simulink model "Supervisory_Control_System"  (R2021a)
settings: Solver=VariableStepAuto  StartTime=0.0  StopTime=10.0  RelTol=1e-3
libraries: simulink x3
settings Model: Creator=shind  LastModifiedBy=shind

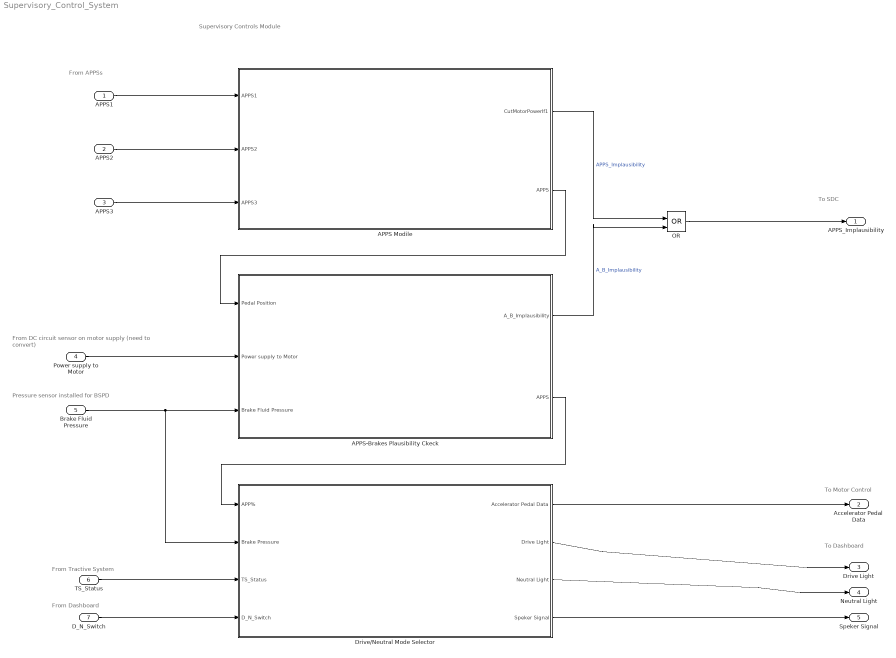
== system Supervisory_Control_System ==
  note: Supervisory Controls Module
  note: From APPSs
  note: To SDC
  note: Pressure sensor installed for
      | BSPD
  note: From DC circuit sensor on motor
      | supply (need to convert)
  note: From Tractive System
  note: From Dashboard
  note: To Motor Control
  note: To Dashboard
  APPS1 : Inport
  APPS2 : Inport  Port=2
  APPS3 : Inport  Port=3
  Power supply to Motor : Inport  Port=4
  Brake Fluid Pressure : Inport  Port=5
  TS_Status : Inport  Port=6
  D_N_Switch : Inport  Port=7
  APPS Modile : Subsystem
  APPS-Brakes Plausibility Ckeck : Subsystem
  Drive/Neutral Mode Selector : Subsystem
  OR : Logic  Operator=OR  IconShape=distinctive  AllPortsSameDT=off  OutDataTypeStr=boolean
  APPS_Implausibility : Outport
  Accelerator Pedal Data : Outport  Port=2
  Drive Light : Outport  Port=3
  Neutral Light : Outport  Port=4
  Speker Signal : Outport  Port=5
  wires:
  APPS2/1 -> APPS Modile/2(APPS2)
  APPS1/1 -> APPS Modile/1(APPS1)
  APPS3/1 -> APPS Modile/3(APPS3)
  APPS Modile/1(CutMotorPowerIf1) -> OR/1  "APPS_Implausibility"
  Power supply to Motor/1 -> APPS-Brakes Plausibility Ckeck/2(Power supply to Motor)
  APPS-Brakes Plausibility Ckeck/1(A_B_Implausibility) -> OR/2  "A_B_Implausibility"
  TS_Status/1 -> Drive/Neutral Mode Selector/3(TS_Status)
  Brake Fluid Pressure/1 -> APPS-Brakes Plausibility Ckeck/3(Brake Fluid Pressure), Drive/Neutral Mode Selector/2(Brake Pressure)
  D_N_Switch/1 -> Drive/Neutral Mode Selector/4(D_N_Switch)
  Drive/Neutral Mode Selector/2(Drive Light) -> Drive Light/1
  Drive/Neutral Mode Selector/3(Neutral Light) -> Neutral Light/1
  Drive/Neutral Mode Selector/1(Accelerator Pedal Data) -> Accelerator Pedal Data/1
  Drive/Neutral Mode Selector/4(Speker Signal) -> Speker Signal/1
  APPS Modile/2(APPS) -> APPS-Brakes Plausibility Ckeck/1(Pedal Position)
  APPS-Brakes Plausibility Ckeck/2(APPS) -> Drive/Neutral Mode Selector/1(APP%)
  OR/1 -> APPS_Implausibility/1

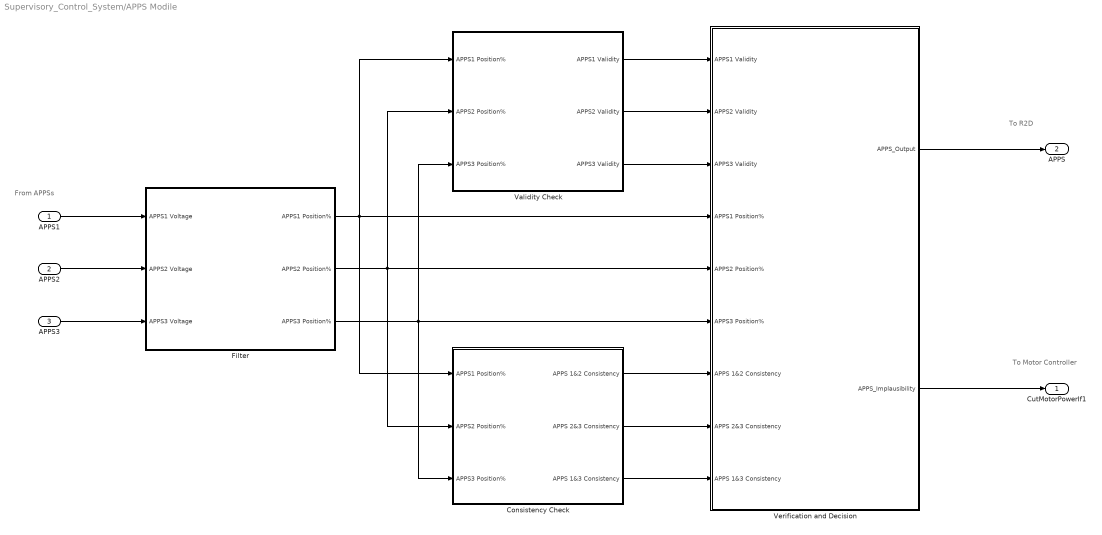
== system Supervisory_Control_System/APPS Modile ==
  note: From APPSs
  note: To Motor Controller
  note: To R2D
  APPS1 : Inport
  APPS2 : Inport  Port=2
  APPS3 : Inport  Port=3
  Consistency Check : Subsystem
  Filter : Subsystem
  Validity Check : Subsystem
  Verification and Decision : Subsystem
  CutMotorPowerIf1 : Outport
  APPS : Outport  Port=2
  wires:
  Verification and Decision/2(APPS_Implausibility) -> CutMotorPowerIf1/1
  APPS2/1 -> Filter/2(APPS2 Voltage)
  Consistency Check/2(APPS 2&3 Consistency) -> Verification and Decision/8(APPS 2&3 Consistency)
  Validity Check/2(APPS2 Validity) -> Verification and Decision/2(APPS2 Validity)
  Filter/1(APPS1 Position%) -> Consistency Check/1(APPS1 Position%), Validity Check/1(APPS1 Position%), Verification and Decision/4(APPS1 Position%)
  Consistency Check/1(APPS 1&2 Consistency) -> Verification and Decision/7(APPS 1&2 Consistency)
  Filter/3(APPS3 Position%) -> Consistency Check/3(APPS3 Position%), Validity Check/3(APPS3 Position%), Verification and Decision/6(APPS3 Position%)
  Validity Check/1(APPS1 Validity) -> Verification and Decision/1(APPS1 Validity)
  Validity Check/3(APPS3 Validity) -> Verification and Decision/3(APPS3 Validity)
  APPS1/1 -> Filter/1(APPS1 Voltage)
  Verification and Decision/1(APPS_Output) -> APPS/1
  APPS3/1 -> Filter/3(APPS3 Voltage)
  Filter/2(APPS2 Position%) -> Consistency Check/2(APPS2 Position%), Validity Check/2(APPS2 Position%), Verification and Decision/5(APPS2 Position%)
  Consistency Check/3(APPS 1&3 Consistency) -> Verification and Decision/9(APPS 1&3 Consistency)

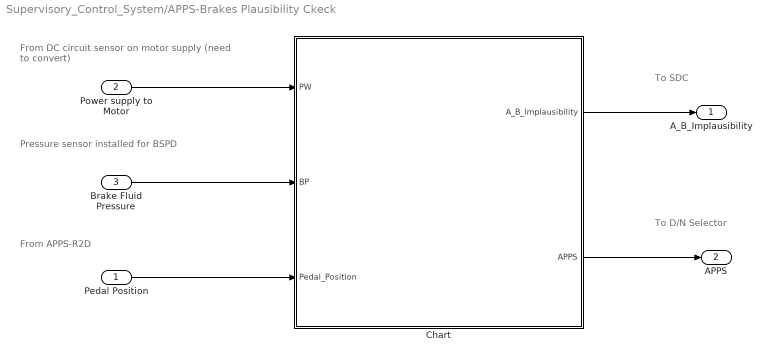
== system Supervisory_Control_System/APPS-Brakes Plausibility Ckeck ==
  note: From DC circuit sensor on motor
      | supply (need to convert)
  note: From APPS-R2D
  note: Pressure sensor installed for
      | BSPD
  note: To SDC
  note: To D/N Selector
  Pedal Position : Inport
  Power supply to Motor : Inport  Port=2
  Brake Fluid Pressure : Inport  Port=3
  Chart : Stateflow chart  TreatAsAtomicUnit=on
  A_B_Implausibility : Outport
  APPS : Outport  Port=2
  wires:
  Power supply to Motor/1 -> Chart/1(PW)
  Brake Fluid Pressure/1 -> Chart/2(BP)
  Pedal Position/1 -> Chart/3(Pedal_Position)
  Chart/1(A_B_Implausibility) -> A_B_Implausibility/1
  Chart/2(APPS) -> APPS/1

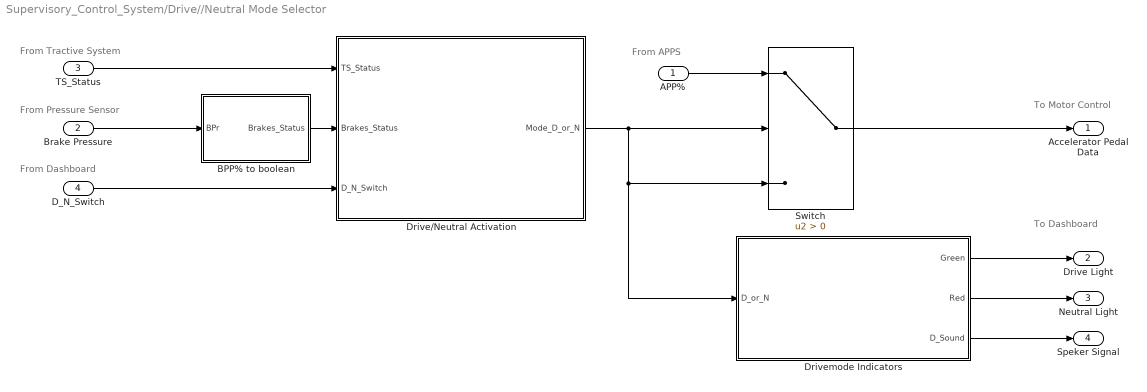
== system Supervisory_Control_System/Drive//Neutral Mode Selector ==
  note: To Motor Control
  note: From Pressure Sensor
  note: From APPS
  note: To Dashboard
  note: From Dashboard
  note: From Tractive System
  APP% : Inport
  Brake Pressure : Inport  Port=2
  TS_Status : Inport  Port=3
  D_N_Switch : Inport  Port=4
  BPP% to boolean : Stateflow chart  TreatAsAtomicUnit=on
  Drive/Neutral Activation : Stateflow chart  TreatAsAtomicUnit=on
  Drivemode Indicators : Stateflow chart  TreatAsAtomicUnit=on
  Switch : Switch  Criteria=u2 > Threshold
  Accelerator Pedal Data : Outport
  Drive Light : Outport  Port=2
  Neutral Light : Outport  Port=3
  Speker Signal : Outport  Port=4
  wires:
  D_N_Switch/1 -> Drive/Neutral Activation/3(D_N_Switch)
  APP%/1 -> Switch/1
  Drive/Neutral Activation/1(Mode_D_or_N) -> Switch/2, Drivemode Indicators/1(D_or_N), Switch/3
  Brake Pressure/1 -> BPP% to boolean/1(BPr)
  BPP% to boolean/1(Brakes_Status) -> Drive/Neutral Activation/2(Brakes_Status)
  Drivemode Indicators/3(D_Sound) -> Speker Signal/1
  Drivemode Indicators/1(Green) -> Drive Light/1
  TS_Status/1 -> Drive/Neutral Activation/1(TS_Status)
  Drivemode Indicators/2(Red) -> Neutral Light/1
  Switch/1 -> Accelerator Pedal Data/1

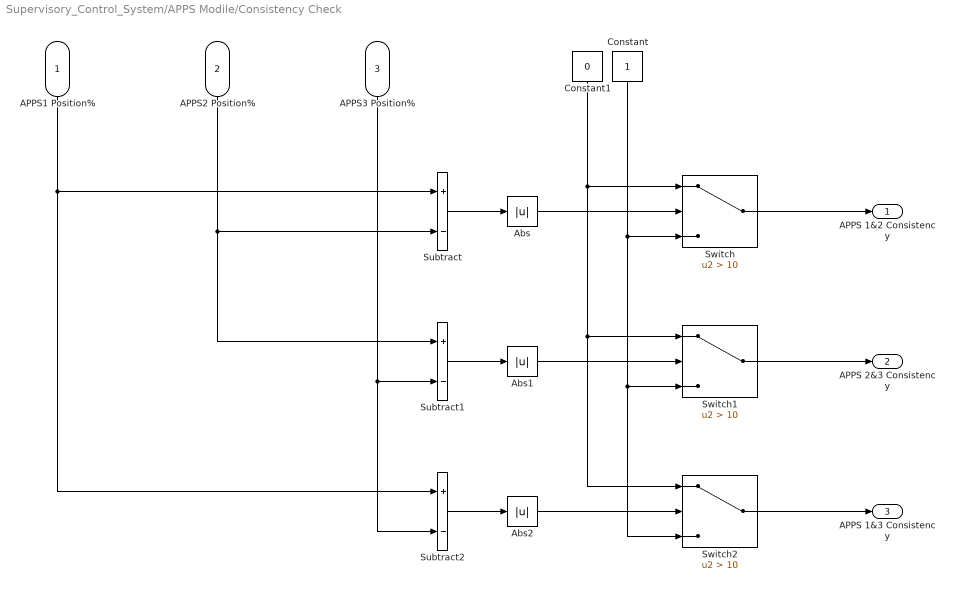
== system Supervisory_Control_System/APPS Modile/Consistency Check ==
  APPS1 Position% : Inport
  APPS2 Position% : Inport  Port=2
  APPS3 Position% : Inport  Port=3
  Abs : Abs
  Abs1 : Abs
  Abs2 : Abs
  Constant : Constant
  Constant1 : Constant  Value=0
  Subtract : Sum  Inputs=+-
  Subtract1 : Sum  Inputs=+-
  Subtract2 : Sum  Inputs=+-
  Switch : Switch  Criteria=u2 > Threshold  Threshold=10
  Switch1 : Switch  Criteria=u2 > Threshold  Threshold=10
  Switch2 : Switch  Criteria=u2 > Threshold  Threshold=10
  APPS 1&2 Consistency : Outport
  APPS 2&3 Consistency : Outport  Port=2
  APPS 1&3 Consistency : Outport  Port=3
  wires:
  Subtract/1 -> Abs/1
  Subtract1/1 -> Abs1/1
  Subtract2/1 -> Abs2/1
  APPS1 Position%/1 -> Subtract/1, Subtract2/1
  APPS2 Position%/1 -> Subtract/2, Subtract1/1
  APPS3 Position%/1 -> Subtract1/2, Subtract2/2
  Abs/1 -> Switch/2
  Constant1/1 -> Switch/1, Switch1/1, Switch2/1
  Constant/1 -> Switch2/3, Switch1/3, Switch/3
  Abs1/1 -> Switch1/2
  Abs2/1 -> Switch2/2
  Switch/1 -> APPS 1&2 Consistency/1
  Switch1/1 -> APPS 2&3 Consistency/1
  Switch2/1 -> APPS 1&3 Consistency/1

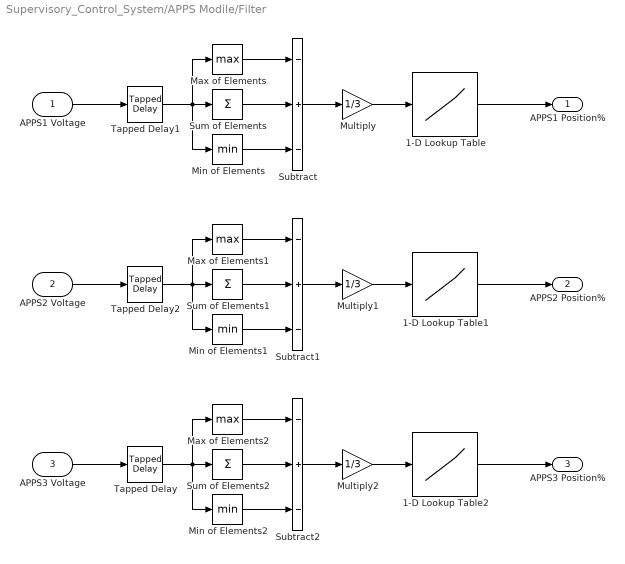
== system Supervisory_Control_System/APPS Modile/Filter ==
  APPS1 Voltage : Inport
  APPS2 Voltage : Inport  Port=2
  APPS3 Voltage : Inport  Port=3
  1-D Lookup Table : Lookup_n-D  NumberOfTableDimensions=1  BreakpointsForDimension1=[-5:5]  Table=tanh([-5:5])  InternalRulePriority=Speed  RndMeth=Simplest  InputSameDT=on
  1-D Lookup Table1 : Lookup_n-D  NumberOfTableDimensions=1  BreakpointsForDimension1=[-5:5]  Table=tanh([-5:5])  InternalRulePriority=Speed  RndMeth=Simplest  InputSameDT=on
  1-D Lookup Table2 : Lookup_n-D  NumberOfTableDimensions=1  BreakpointsForDimension1=[-5:5]  Table=tanh([-5:5])  InternalRulePriority=Speed  RndMeth=Simplest  InputSameDT=on
  Max of Elements : MinMax  Function=max
  Max of Elements1 : MinMax  Function=max
  Max of Elements2 : MinMax  Function=max
  Min of Elements : MinMax
  Min of Elements1 : MinMax
  Min of Elements2 : MinMax
  Multiply : Gain  Gain=1/3
  Multiply1 : Gain  Gain=1/3
  Multiply2 : Gain  Gain=1/3
  Subtract : Sum  Inputs=-+-
  Subtract1 : Sum  Inputs=-+-
  Subtract2 : Sum  Inputs=-+-
  Sum of Elements : Sum  Inputs=+
  Sum of Elements1 : Sum  Inputs=+
  Sum of Elements2 : Sum  Inputs=+
  Tapped Delay : simulink/Discrete/Tapped Delay  vinit=0.0  samptime=-1  NumDelays=5  DelayOrder=Oldest  includeCurrent=off
  Tapped Delay1 : simulink/Discrete/Tapped Delay  vinit=0.0  samptime=-1  NumDelays=5  DelayOrder=Oldest  includeCurrent=off
  Tapped Delay2 : simulink/Discrete/Tapped Delay  vinit=0.0  samptime=-1  NumDelays=5  DelayOrder=Oldest  includeCurrent=off
  APPS1 Position% : Outport
  APPS2 Position% : Outport  Port=2
  APPS3 Position% : Outport  Port=3
  wires:
  Multiply2/1 -> 1-D Lookup Table2/1
  1-D Lookup Table2/1 -> APPS3 Position%/1
  Multiply/1 -> 1-D Lookup Table/1
  APPS2 Voltage/1 -> Tapped Delay2/1
  Max of Elements/1 -> Subtract/1
  Subtract2/1 -> Multiply2/1
  Sum of Elements/1 -> Subtract/2
  Max of Elements2/1 -> Subtract2/1
  Sum of Elements2/1 -> Subtract2/2
  Sum of Elements1/1 -> Subtract1/2
  Subtract1/1 -> Multiply1/1
  Subtract/1 -> Multiply/1
  Min of Elements1/1 -> Subtract1/3
  1-D Lookup Table1/1 -> APPS2 Position%/1
  Min of Elements2/1 -> Subtract2/3
  APPS1 Voltage/1 -> Tapped Delay1/1
  Max of Elements1/1 -> Subtract1/1
  Min of Elements/1 -> Subtract/3
  APPS3 Voltage/1 -> Tapped Delay/1
  Multiply1/1 -> 1-D Lookup Table1/1
  Tapped Delay2/1 -> Sum of Elements1/1, Max of Elements1/1, Min of Elements1/1
  Tapped Delay1/1 -> Max of Elements/1, Sum of Elements/1, Min of Elements/1
  Tapped Delay/1 -> Sum of Elements2/1, Max of Elements2/1, Min of Elements2/1
  1-D Lookup Table/1 -> APPS1 Position%/1

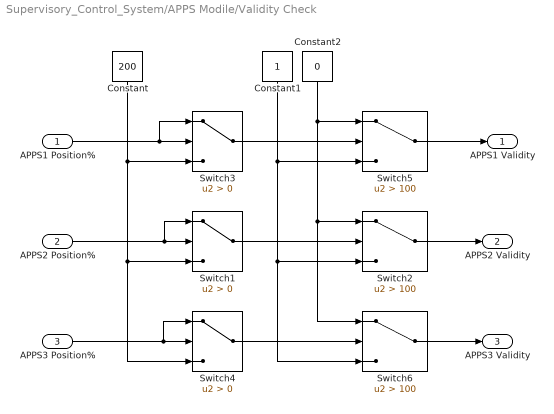
== system Supervisory_Control_System/APPS Modile/Validity Check ==
  APPS1 Position% : Inport
  APPS2 Position% : Inport  Port=2
  APPS3 Position% : Inport  Port=3
  Constant : Constant  Value=200
  Constant1 : Constant
  Constant2 : Constant  Value=0
  Switch1 : Switch  Criteria=u2 > Threshold
  Switch2 : Switch  Criteria=u2 > Threshold  Threshold=100
  Switch3 : Switch  Criteria=u2 > Threshold
  Switch4 : Switch  Criteria=u2 > Threshold
  Switch5 : Switch  Criteria=u2 > Threshold  Threshold=100
  Switch6 : Switch  Criteria=u2 > Threshold  Threshold=100
  APPS1 Validity : Outport
  APPS2 Validity : Outport  Port=2
  APPS3 Validity : Outport  Port=3
  wires:
  Switch5/1 -> APPS1 Validity/1
  APPS1 Position%/1 -> Switch3/1, Switch3/2
  Switch3/1 -> Switch5/2
  Switch1/1 -> Switch2/2
  APPS2 Position%/1 -> Switch1/2, Switch1/1
  Switch2/1 -> APPS2 Validity/1
  Switch6/1 -> APPS3 Validity/1
  APPS3 Position%/1 -> Switch4/1, Switch4/2
  Switch4/1 -> Switch6/2
  Constant/1 -> Switch3/3, Switch1/3, Switch4/3
  Constant1/1 -> Switch6/3, Switch2/3, Switch5/3
  Constant2/1 -> Switch6/1, Switch2/1, Switch5/1

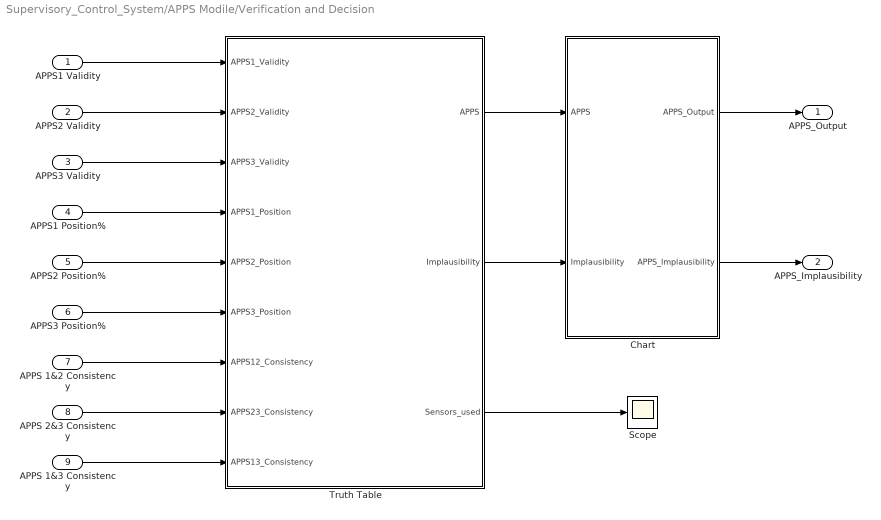
== system Supervisory_Control_System/APPS Modile/Verification and Decision ==
  APPS1 Validity : Inport
  APPS2 Validity : Inport  Port=2
  APPS3 Validity : Inport  Port=3
  APPS1 Position% : Inport  Port=4
  APPS2 Position% : Inport  Port=5
  APPS3 Position% : Inport  Port=6
  APPS 1&2 Consistency : Inport  Port=7
  APPS 2&3 Consistency : Inport  Port=8
  APPS 1&3 Consistency : Inport  Port=9
  Chart : Stateflow chart  TreatAsAtomicUnit=on
  Scope : Scope
  Truth Table : Truth Table  TreatAsAtomicUnit=on
  APPS_Output : Outport
  APPS_Implausibility : Outport  Port=2
  wires:
  APPS1 Validity/1 -> Truth Table/1(APPS1_Validity)
  APPS2 Validity/1 -> Truth Table/2(APPS2_Validity)
  APPS3 Validity/1 -> Truth Table/3(APPS3_Validity)
  APPS1 Position%/1 -> Truth Table/4(APPS1_Position)
  APPS2 Position%/1 -> Truth Table/5(APPS2_Position)
  APPS3 Position%/1 -> Truth Table/6(APPS3_Position)
  APPS 1&2 Consistency/1 -> Truth Table/7(APPS12_Consistency)
  APPS 2&3 Consistency/1 -> Truth Table/8(APPS23_Consistency)
  APPS 1&3 Consistency/1 -> Truth Table/9(APPS13_Consistency)
  Truth Table/3(Sensors_used) -> Scope/1
  Truth Table/1(APPS) -> Chart/1(APPS)
  Truth Table/2(Implausibility) -> Chart/2(Implausibility)
  Chart/1(APPS_Output) -> APPS_Output/1
  Chart/2(APPS_Implausibility) -> APPS_Implausibility/1

== stateflow chart Supervisory_Control_System/Drive//Neutral Mode Selector/Drivemode Indicators ==
  state Neutral
    entry:
    Red=1;
    Green=0;
  state Drive
    entry:
    Red=0;
    Green=1;
    state sound_start
      entry:
      D_Sound=1;
    state sound_stop
      entry:
      D_Sound=0;
    (default) -> sound_start
    sound_start -> sound_stop : after(2,sec)
  (default) -> Neutral
  Neutral -> Drive : [D_or_N==1]
  Drive -> Neutral : [D_or_N==0]
  data: D_or_N input; Green output; Red output; D_Sound output

== stateflow chart Supervisory_Control_System/APPS-Brakes Plausibility Ckeck/Chart ==
  state Normal
    entry:
    A_B_Implausibility=0;
    APPS=Pedal_Position;
  state APPS_Brake_Implausible
    entry:
    A_B_Implausibility=1;
    APPS=0;
  state Time_Check
  (default) -> Normal
  Normal -> Time_Check : [BP>=30 && PW>=5000]
  Time_Check -> APPS_Brake_Implausible [order 1] : after(500,msec)
  Time_Check -> Normal [order 2] : [BP<30 || PW<5000]
  APPS_Brake_Implausible -> Normal : [Pedal_Position==0]
  data: A_B_Implausibility output; PW input; BP input; Pedal_Position input; APPS output

== matlab function Supervisory_Control_System/APPS Modile/Verification and Decision/Truth Table ==
  data: APPS1_Validity input; APPS2_Validity input double; APPS3_Validity input double; APPS1_Position input double; APPS2_Position input double; APPS3_Position input double; APPS12_Consistency input double; APPS23_Consistency input double; APPS13_Consistency input double; APPS output double; Implausibility output double; Sensors_used output double
function [APPS, Implausibility, Sensors_used] = fcn(APPS1_Validity, APPS2_Validity, APPS3_Validity, APPS1_Position, APPS2_Position, APPS3_Position, APPS12_Consistency, APPS23_Consistency, APPS13_Consistency)

aVarTruthTableCondition_1 = false;
aVarTruthTableCondition_2 = false;
aVarTruthTableCondition_3 = false;
aVarTruthTableCondition_4 = false;
aVarTruthTableCondition_5 = false;
aVarTruthTableCondition_6 = false;


% 1 Validity

aVarTruthTableCondition_1 = logical(APPS1_Validity==1);

% 2 Validity

aVarTruthTableCondition_2 = logical(APPS2_Validity==1);

% 3 Validity

aVarTruthTableCondition_3 = logical(APPS3_Validity==1);

% 12 Consistency

aVarTruthTableCondition_4 = logical(APPS12_Consistency==1);

% 23 Consistency

aVarTruthTableCondition_5 = logical(APPS23_Consistency==1);

% 13 Consistency

aVarTruthTableCondition_6 = logical(APPS13_Consistency==1);

if (aVarTruthTableCondition_1 && aVarTruthTableCondition_2 && aVarTruthTableCondition_3 && aVarTruthTableCondition_4 && aVarTruthTableCondition_5 && aVarTruthTableCondition_6)
    aFcnTruthTableAction_1();
elseif (aVarTruthTableCondition_1 && aVarTruthTableCondition_2 && ~aVarTruthTableCondition_3 && aVarTruthTableCondition_4)
    aFcnTruthTableAction_2();
elseif (aVarTruthTableCondition_1 && aVarTruthTableCondition_2 && aVarTruthTableCondition_3 && aVarTruthTableCondition_4 && ~aVarTruthTableCondition_5)
    aFcnTruthTableAction_2();
elseif (aVarTruthTableCondition_1 && aVarTruthTableCondition_2 && aVarTruthTableCondition_3 && aVarTruthTableCondition_4 && ~aVarTruthTableCondition_6)
    aFcnTruthTableAction_2();
elseif (~aVarTruthTableCondition_1 && aVarTruthTableCondition_2 && aVarTruthTableCondition_3 && aVarTruthTableCondition_5)
    aFcnTruthTableAction_3();
elseif (aVarTruthTableCondition_1 && aVarTruthTableCondition_2 && aVarTruthTableCondition_3 && ~aVarTruthTableCondition_4 && aVarTruthTableCondition_5)
    aFcnTruthTableAction_3();
elseif (aVarTruthTableCondition_1 && ~aVarTruthTableCondition_2 && aVarTruthTableCondition_3 && aVarTruthTableCondition_6)
    aFcnTruthTableAction_4();
elseif (aVarTruthTableCondition_1 && aVarTruthTableCondition_2 && aVarTruthTableCondition_3 && ~aVarTruthTableCondition_4 && ~aVarTruthTableCondition_5 && aVarTruthTableCondition_6)
    aFcnTruthTableAction_4();
elseif (~aVarTruthTableCondition_1 && ~aVarTruthTableCondition_2)
    aFcnTruthTableAction_5();
elseif (~aVarTruthTableCondition_2 && ~aVarTruthTableCondition_3)
    aFcnTruthTableAction_5();
elseif (~aVarTruthTableCondition_1 && ~aVarTruthTableCondition_3)
    aFcnTruthTableAction_5();
elseif (aVarTruthTableCondition_1 && aVarTruthTableCondition_2 && aVarTruthTableCondition_3 && ~aVarTruthTableCondition_4 && ~aVarTruthTableCondition_5 && ~aVarTruthTableCondition_6)
    aFcnTruthTableAction_5();
elseif (aVarTruthTableCondition_1 && aVarTruthTableCondition_2 && ~aVarTruthTableCondition_3 && ~aVarTruthTableCondition_4)
    aFcnTruthTableAction_5();
elseif (~aVarTruthTableCondition_1 && aVarTruthTableCondition_2 && aVarTruthTableCondition_3 && ~aVarTruthTableCondition_5)
    aFcnTruthTableAction_5();
else % Default
    aFcnTruthTableAction_5();
end

function aFcnTruthTableAction_1()

% All 3 sensors working and will be used

APPS=((APPS1_Position+APPS2_Position+APPS3_Position)/3);
Implausibility=0;
Sensors_used=6;

function aFcnTruthTableAction_2()

% Sensors 12 will be used

APPS=((APPS1_Position+APPS2_Position)/2);
Implausibility=0;
Sensors_used=3;

function aFcnTruthTableAction_3()

% Sensors 23 wil be used

APPS=((APPS2_Position+APPS3_Position)/2);
Implausibility=0;
Sensors_used=5;

function aFcnTruthTableAction_4()

% Sensors 13 wil be used

APPS=((APPS1_Position+APPS3_Position)/2);
Implausibility=0;
Sensors_used=4;

function aFcnTruthTableAction_5()

% No pair of sensors usable and implausibility should occure in 100ms

APPS=((APPS1_Position+APPS2_Position+APPS3_Position)/3);
Implausibility=1;
Sensors_used=0;

== stateflow chart Supervisory_Control_System/APPS Modile/Verification and Decision/Chart ==
  state Normal
    entry:
    APPS_Implausibility=0;
    APPS_Output=APPS;
  state Implausible_Declaration
    entry:
    APPS_Implausibility=1;
    APPS_Output=0;
  state Time_Check
  (default) -> Normal
  Normal -> Time_Check : [Implausibility==1]
  Time_Check -> Implausible_Declaration [order 2] : after(100,msec)
  Time_Check -> Normal [order 1] : [Implausibility==0]
  data: APPS_Output output; APPS_Implausibility output; APPS input; Implausibility input

== stateflow chart Supervisory_Control_System/Drive//Neutral Mode Selector/BPP% to boolean ==
  state Brakes_not_actuated
    entry:
    Brakes_Status==0;
  state Brakes_actuated
    entry:
    Brakes_Status==1;
  (default) -> Brakes_not_actuated
  Brakes_not_actuated -> Brakes_actuated : [BPr>20]
  Brakes_actuated -> Brakes_not_actuated : [BPr<20]
  data: BPr input; Brakes_Status output =00

== stateflow chart Supervisory_Control_System/Drive//Neutral Mode Selector/Drive//Neutral Activation ==
  state Neutral
    entry:
    Mode_D_or_N=0;
  state Consistant_action_check_for_D
  state Drive
    entry:
    Mode_D_or_N=1;
  state Consistant_action_check_for_N
  (default) -> Neutral
  Neutral -> Consistant_action_check_for_D : [Brakes_Status==1 && TS_Status==1 && D_N_Switch==1]
  Consistant_action_check_for_D -> Drive [order 2] : after(1,sec)
  Consistant_action_check_for_D -> Neutral [order 1] : [Brakes_Status==0 || TS_Status==0 || D_N_Switch==0]
  Drive -> Neutral [order 1] : [TS_Status==0]
  Drive -> Consistant_action_check_for_N [order 2] : [Brakes_Status==1 && D_N_Switch==1]
  Consistant_action_check_for_N -> Neutral [order 2] : after(500,msec)
  Consistant_action_check_for_N -> Drive [order 1] : [Brakes_Status==0 || D_N_Switch==0]
  data: TS_Status input; Brakes_Status input; D_N_Switch input; Mode_D_or_N output
